simulink model "Tutorial_Simulink_4"  (R2024a)
settings: Solver=VariableStepAuto  StartTime=0.0  StopTime=10.0  RelTol=1e-3
settings Model: Creator=gzipprich  LastModifiedBy=gzipprich

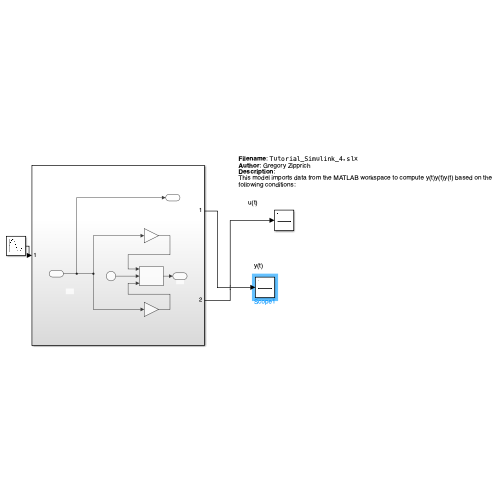
[thumbnail: Simulink's stored preview of the top-level diagram]
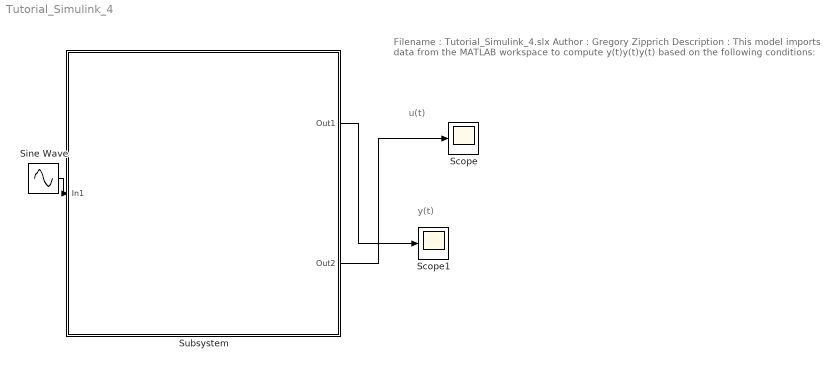
== system Tutorial_Simulink_4 ==
  note: y(t)
  note: u(t)
  note: Filename : Tutorial_Simulink_4.slx
      | Author : Gregory Zipprich
      | Description :
      | This model imports data from the MATLAB workspace to compute y(t)y(t)y(t) based on the following conditions:
  Scope : Scope
  Scope1 : Scope
  Sine Wave : Sin  SampleTime=0
  Subsystem : Subsystem
  wires:
  Sine Wave/1 -> Subsystem/1(In1)
  Subsystem/2(Out2) -> Scope/1
  Subsystem/1(Out1) -> Scope1/1

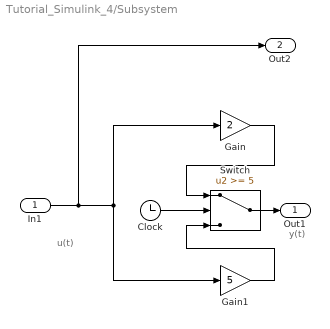
== system Tutorial_Simulink_4/Subsystem ==
  note: y(t)
  note: u(t)
  In1 : Inport
  Clock : Clock
  Gain : Gain  Gain=2
  Gain1 : Gain  Gain=5
  Switch : Switch  Threshold=5  SaturateOnIntegerOverflow=off  InputSameDT=off
  Out1 : Outport
  Out2 : Outport  Port=2
  wires:
  Clock/1 -> Switch/2
  Switch/1 -> Out1/1
  Gain1/1 -> Switch/3
  In1/1 -> Out2/1, Gain1/1, Gain/1
  Gain/1 -> Switch/1
